simulink model "BF_Q2"  (R2025b)
settings: Solver=VariableStepAuto  StartTime=0.0  StopTime=10.0  RelTol=1e-3
values from neighbouring files (symbols this model uses):
  Gb = 92    [Dev_04_M.m]
  Ib = 7.3    [Dev_04_M.m]
  Kd = 0.01    [Dev_04_M.m]
  Ki = 0.1    [Dev_04_M.m]
  Kp = 5    [Dev_04_M.m]
  n = 0.3    [Dev_04_M.m]
  p1 = 0.03    [Dev_04_M.m]
  p2 = 0.02    [Dev_04_M.m]
  p3 = 1.06*(10^-5)    (= 1.06e-05)    [Dev_04_M.m]
  x0 = [92; 0; 7.3; 0]    [Dev_04_M.m]
settings Model: Creator=Louis  LastModifiedBy=diegoalfonsocosta

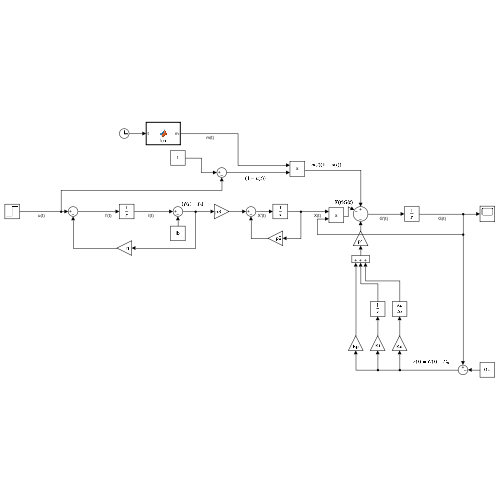
[thumbnail: Simulink's stored preview of the top-level diagram]
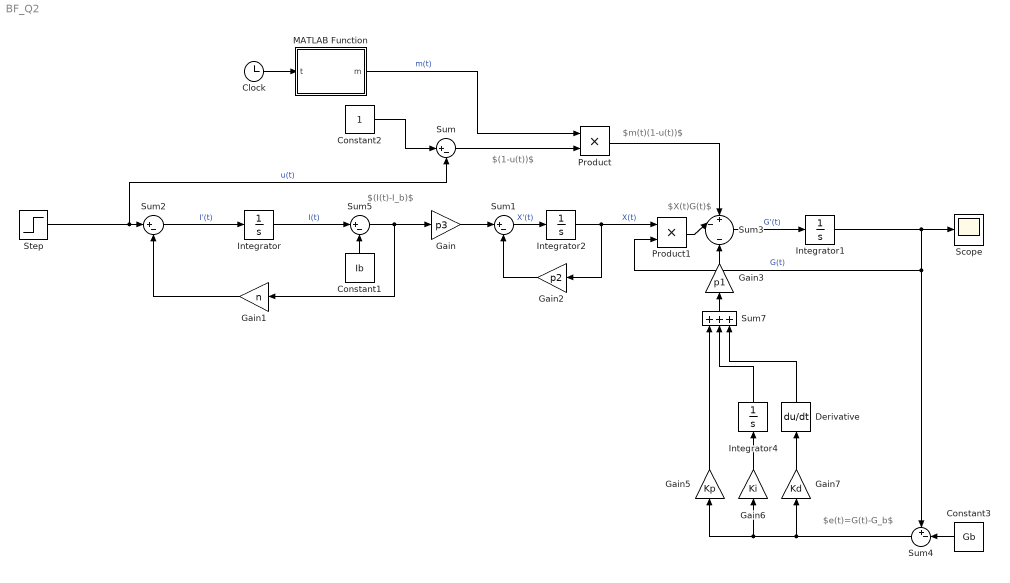
== system BF_Q2 ==
  note: $m(t)(1-u(t))$
  note: $X(t)G(t)$
  note: $(I(t)-I_b)$
  note: $e(t)=G(t)-G_b$
  note: $(1-u(t))$
  Clock : Clock
  Constant1 : Constant  Value=Ib
  Constant2 : Constant
  Constant3 : Constant  Value=Gb
  Derivative : Derivative
  Gain : Gain  Gain=p3
  Gain1 : Gain  Gain=n
  Gain2 : Gain  Gain=p2
  Gain3 : Gain  Gain=p1
  Gain5 : Gain  Gain=Kp
  Gain6 : Gain  Gain=Ki
  Gain7 : Gain  Gain=Kd
  Integrator : Integrator  InitialCondition=x0(3)
  Integrator1 : Integrator  InitialCondition=x0(1)
  Integrator2 : Integrator  InitialCondition=x0(2)
  Integrator4 : Integrator
  MATLAB Function : MATLAB Function  TreatAsAtomicUnit=on
  Product : Product
  Product1 : Product
  Scope : Scope
      settings: ActiveDisplayYMinimum=-1  ActiveDisplayYMaximum=1  DataLoggingVariableName=GBF_Q2  DataLoggingSaveFormat=Array
  Step : Step  Time=0  After=2  SampleTime=0
  Sum{,1..2,5} (4 alike) : Sum  Inputs=|+-
  Sum3 : Sum  Inputs=+-|-
  Sum4 : Sum  Inputs=+-|
  Sum7 : Sum  Inputs=+++
  wires:
  MATLAB Function/1(m) -> Product/1  "m(t)"
  Product/1 -> Sum3/1
  Gain6/1 -> Integrator4/1
  Constant1/1 -> Sum5/2
  Integrator4/1 -> Sum7/2
  Gain/1 -> Sum1/1
  Constant3/1 -> Sum4/2
  Sum5/1 -> Gain1/1, Gain/1
  Integrator1/1 -> Scope/1, Product1/2, Sum4/1  "G(t)"
  Derivative/1 -> Sum7/3
  Sum2/1 -> Integrator/1  "I'(t)"
  Gain3/1 -> Sum3/3
  Sum7/1 -> Gain3/1
  Integrator2/1 -> Product1/1, Gain2/1  "X(t)"
  Sum1/1 -> Integrator2/1  "X'(t)"
  Gain5/1 -> Sum7/1
  Sum3/1 -> Integrator1/1  "G'(t)"
  Sum4/1 -> Gain7/1, Gain6/1, Gain5/1
  Gain7/1 -> Derivative/1
  Integrator/1 -> Sum5/1  "I(t)"
  Sum/1 -> Product/2
  Constant2/1 -> Sum/1
  Step/1 -> Sum/2, Sum2/1  "u(t)"
  Gain1/1 -> Sum2/2
  Product1/1 -> Sum3/2
  Gain2/1 -> Sum1/2
  Clock/1 -> MATLAB Function/1(t)

== matlab function BF_Q2/MATLAB Function ==
  data: t input; m output
function m = fcn(t)

if (t >= 0 && t <= 5)
    m = 5*1;

else
    m = 0;
end
